simulink model "main_model"  (R2022a)
settings: Solver=VariableStepAuto  StartTime=0.0  StopTime=10.0  RelTol=1e-3
libraries: visionsources x2
settings Model: Creator=DASARI SUDHEERA  LastModifiedBy=DASARI SUDHEERA

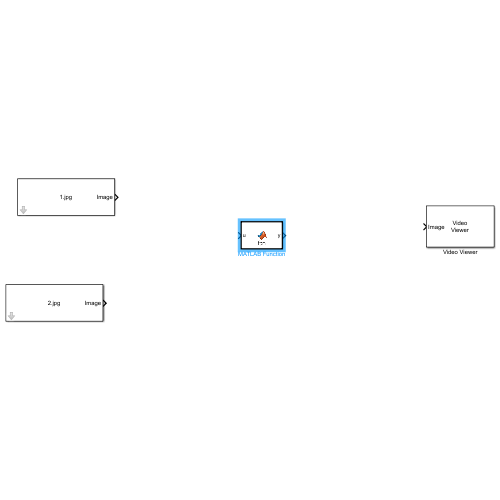
[thumbnail: Simulink's stored preview of the top-level diagram]
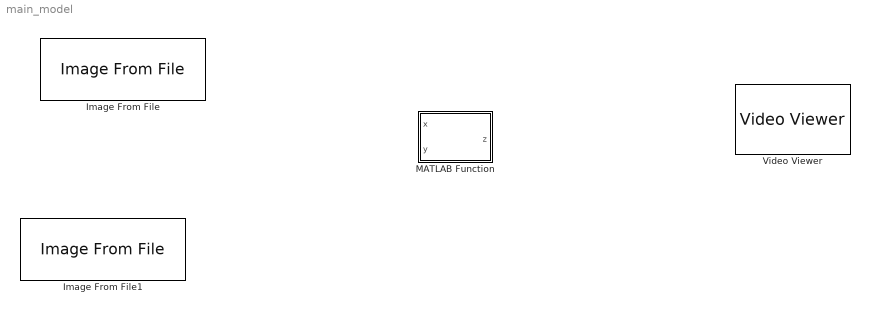
== system main_model ==
  Image From File : visionsources/Image From File  Tag=vipblks_nd  FileName=C:\photos\s1\1.jpg  Ts=inf  imagePorts=One multidimensional signal  OutPortLabels=R|G|B  ImageDataType=Inherit from input image  sdImageDataType=uint(8)  Signed=on  WordLength=16  FractionLengthMode=User-defined  FractionLength=15
  Image From File1 : visionsources/Image From File  Tag=vipblks_nd  FileName=C:\photos\s1\2.jpg  Ts=inf  imagePorts=One multidimensional signal  OutPortLabels=R|G|B  ImageDataType=Inherit from input image  sdImageDataType=uint(8)  Signed=on  WordLength=16  FractionLengthMode=User-defined  FractionLength=15
  MATLAB Function : MATLAB Function  TreatAsAtomicUnit=on
  Video Viewer : VideoViewer  FigPos=[2041 741 418 304]

== matlab function main_model/MATLAB Function ==
  data: x input; z output; y input
function z = fcn(x,y)
g=size(x);
y=imresize(y[g(1)g(2)]);
figure;
z=(x=y);
